simulink model "Feedforward_Control"  (R2025b)
settings: Solver=VariableStepAuto  StartTime=0.0  StopTime=10.0  RelTol=1e-3
settings Model: Creator=koryh  LastModifiedBy=koryh

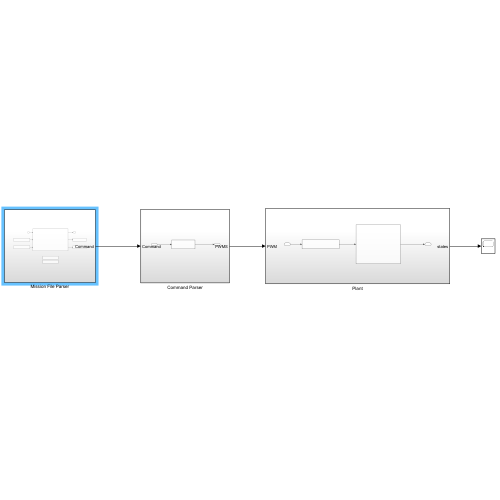
[thumbnail: Simulink's stored preview of the top-level diagram]
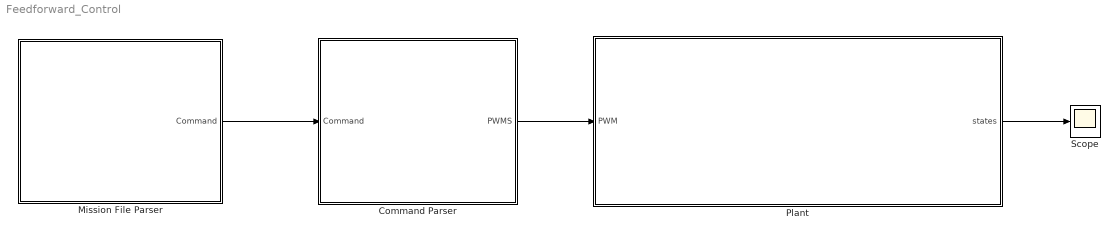
== system Feedforward_Control ==
  Command Parser : Subsystem
  Mission File Parser : Subsystem
  Plant : Subsystem
  Scope : Scope
  wires:
  Mission File Parser/1(Command) -> Command Parser/1(Command)
  Command Parser/1(PWMS) -> Plant/1(PWM)
  Plant/1(states) -> Scope/1

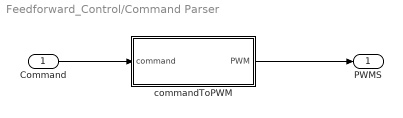
== system Feedforward_Control/Command Parser ==
  Command : Inport
  commandToPWM : MATLAB Function  TreatAsAtomicUnit=on
  PWMS : Outport
  wires:
  commandToPWM/1(PWM) -> PWMS/1
  Command/1 -> commandToPWM/1(command)

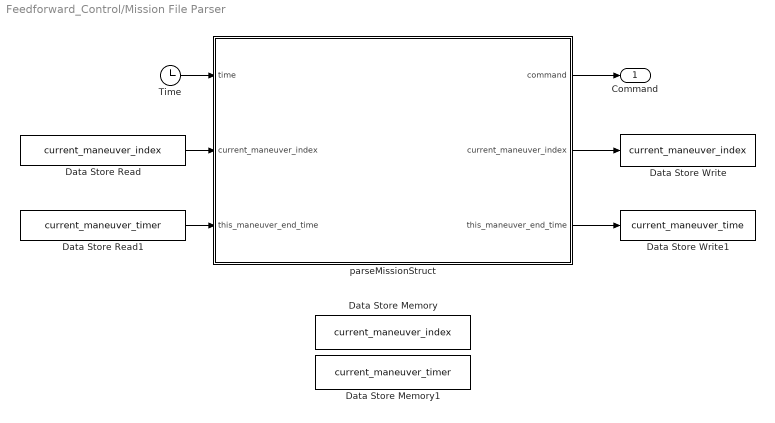
== system Feedforward_Control/Mission File Parser ==
  Data Store Memory : DataStoreMemory  DataStoreName=current_maneuver_index  WriteAfterWriteMsg=warning  InitialValue=1  ShowAdditionalParam=off
  Data Store Memory1 : DataStoreMemory  DataStoreName=current_maneuver_timer  WriteAfterWriteMsg=warning  ShowAdditionalParam=off
  Data Store Read : DataStoreRead  DataStoreName=current_maneuver_index  IndexOptions=Index vector (dialog)  Indices=1  OutputSizes=1
  Data Store Read1 : DataStoreRead  DataStoreName=current_maneuver_timer  IndexOptions=Index vector (dialog)  Indices=1  OutputSizes=1
  Data Store Write : DataStoreWrite  DataStoreName=current_maneuver_index  IndexOptions=Index vector (dialog)  Indices=1  OutputSizes=1
  Data Store Write1 : DataStoreWrite  DataStoreName=current_maneuver_time  IndexOptions=Index vector (dialog)  Indices=1  OutputSizes=1
  Time : Clock
  parseMissionStruct : MATLAB Function  TreatAsAtomicUnit=on
  Command : Outport
  wires:
  Time/1 -> parseMissionStruct/1(time)
  parseMissionStruct/1(command) -> Command/1
  Data Store Read/1 -> parseMissionStruct/2("current_maneuver_index ")
  Data Store Read1/1 -> parseMissionStruct/3("this_maneuver_end_time ")
  parseMissionStruct/2(current_maneuver_index) -> Data Store Write/1
  parseMissionStruct/3(this_maneuver_end_time) -> Data Store Write1/1

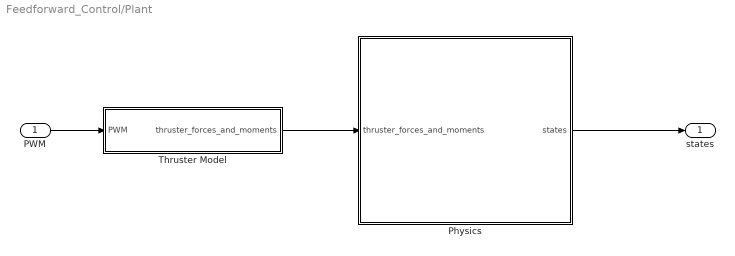
== system Feedforward_Control/Plant ==
  PWM : Inport
  Physics : Subsystem
  Thruster Model : Subsystem
  states : Outport
  wires:
  PWM/1 -> Thruster Model/1(PWM)
  Thruster Model/1(thruster_forces_and_moments) -> Physics/1(thruster_forces_and_moments)
  Physics/1(states) -> states/1

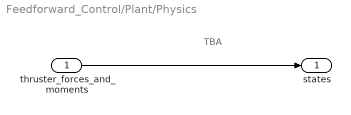
== system Feedforward_Control/Plant/Physics ==
  note: TBA
  thruster_forces_and_moments : Inport
  states : Outport
  wires:
  thruster_forces_and_moments/1 -> states/1

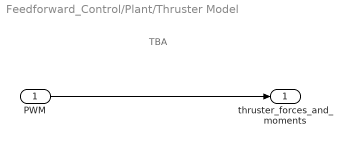
== system Feedforward_Control/Plant/Thruster Model ==
  note: TBA
  PWM : Inport
  thruster_forces_and_moments : Outport
  wires:
  PWM/1 -> thruster_forces_and_moments/1

== matlab function Feedforward_Control/Command Parser/commandToPWM ==
  data: command input; PWM output
function PWM = fcn(command)

PWM = command2PWM(command); %see utils

== matlab function Feedforward_Control/Mission File Parser/parseMissionStruct ==
  data: mission_struct parameter; command output; time input; current_maneuver_index input; this_maneuver_end_time input; current_maneuver_index output; this_maneuver_end_time output
function [command, current_maneuver_index, this_maneuver_end_time] = ...
    fcn(mission_struct,time,current_maneuver_index,this_maneuver_end_time)

[command, current_maneuver_index, this_maneuver_end_time] = ...
    parseMissionStruct(mission_struct,time,current_maneuver_index,...
    this_maneuver_end_time); %see utils
